simulink model "Lab_04_Task03"  (R2015a)
settings: Solver=ode45  StartTime=0.0  StopTime=10.0  RelTol=1e-3
libraries: cstblocks x7
settings Model: Creator=Amir  LastModifiedBy=Amir

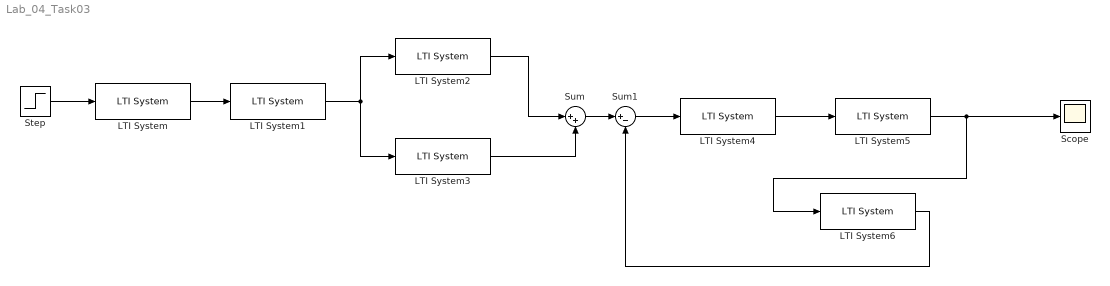
== system Lab_04_Task03 ==
  LTI System : cstblocks/LTI System  sys=tf(1,[1 1])  IC=[]
  LTI System1 : cstblocks/LTI System  sys=tf(1,[1 3])  IC=[]
  LTI System2 : cstblocks/LTI System  sys=tf([1 3],[1 5])  IC=[]
  LTI System3 : cstblocks/LTI System  sys=tf(1,[1 1])  IC=[]
  LTI System4 : cstblocks/LTI System  sys=tf(1,[1 3])  IC=[]
  LTI System5 : cstblocks/LTI System  sys=tf(1,[1 1])  IC=[]
  LTI System6 : cstblocks/LTI System  sys=tf([1 3],[1 5])  IC=[]
  Scope : Scope
  Step : Step  SampleTime=0
  Sum : Sum  Inputs=|++
  Sum1 : Sum  Inputs=|+-
  wires:
  Step/1 -> LTI System/1
  LTI System/1 -> LTI System1/1
  LTI System1/1 -> LTI System3/1, LTI System2/1
  LTI System3/1 -> Sum/2
  LTI System2/1 -> Sum/1
  Sum/1 -> Sum1/1
  LTI System4/1 -> LTI System5/1
  Sum1/1 -> LTI System4/1
  LTI System6/1 -> Sum1/2
  LTI System5/1 -> LTI System6/1, Scope/1
